simulink model "T_transmitter"  (R2023b)
settings: Solver=ode45  StartTime=0.0  StopTime=10.0  RelTol=1e-3
undefined symbols (not defined in the file or in its folder): I
libraries: simulink x1
settings Model: Creator=86186  LastModifiedBy=86186

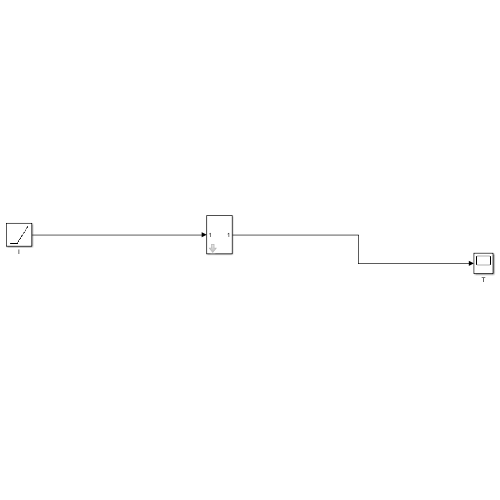
[thumbnail: Simulink's stored preview of the top-level diagram]
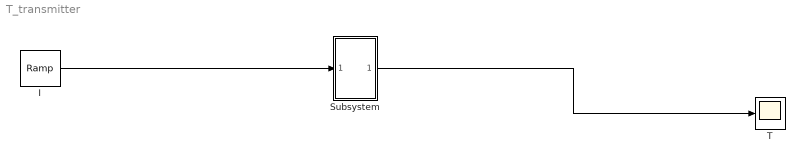
== system T_transmitter ==
  I : simulink/Sources/Ramp  slope=I  start=0  InitialOutput=0
  Subsystem : Subsystem  mask{Imin=0, Imax=40, Tmin=30, Tmax=100}
      mask prompts: Imin "最小电流"; Imax "最大电流"; Tmin "最小温度"; Tmax "最大温度"
      mask DialogControl ParameterGroupVar Prompt: 参数
  T : Scope
  wires:
  I/1 -> Subsystem/1(In1)
  Subsystem/1(Out1) -> T/1

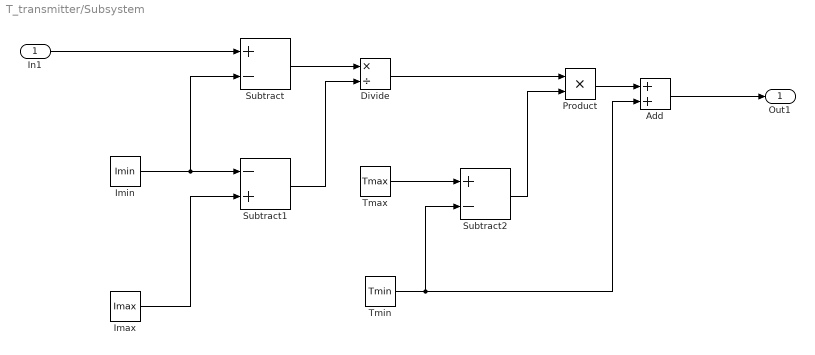
== system T_transmitter/Subsystem ==
  In1 : Inport
  Add : Sum
  Divide : Product  Inputs=*/
  Imax : Constant  Value=Imax
  Imin : Constant  Value=Imin
  Product : Product
  Subtract : Sum  Inputs=+-
  Subtract1 : Sum  Inputs=-+
  Subtract2 : Sum  Inputs=+-
  Tmax : Constant  Value=Tmax
  Tmin : Constant  Value=Tmin
  Out1 : Outport
  wires:
  Subtract/1 -> Divide/1
  Tmin/1 -> Add/2, Subtract2/2
  In1/1 -> Subtract/1
  Subtract2/1 -> Product/2
  Tmax/1 -> Subtract2/1
  Imin/1 -> Subtract1/1, Subtract/2
  Imax/1 -> Subtract1/2
  Subtract1/1 -> Divide/2
  Product/1 -> Add/1
  Divide/1 -> Product/1
  Add/1 -> Out1/1
